simulink model "mode_glissant"  (R2016b)
settings: Solver=FixedStepAuto  StartTime=0.0  StopTime=10.0  FixedStep=.1  RelTol=1e-3
settings Model: Creator=vanou  LastModifiedBy=vanou

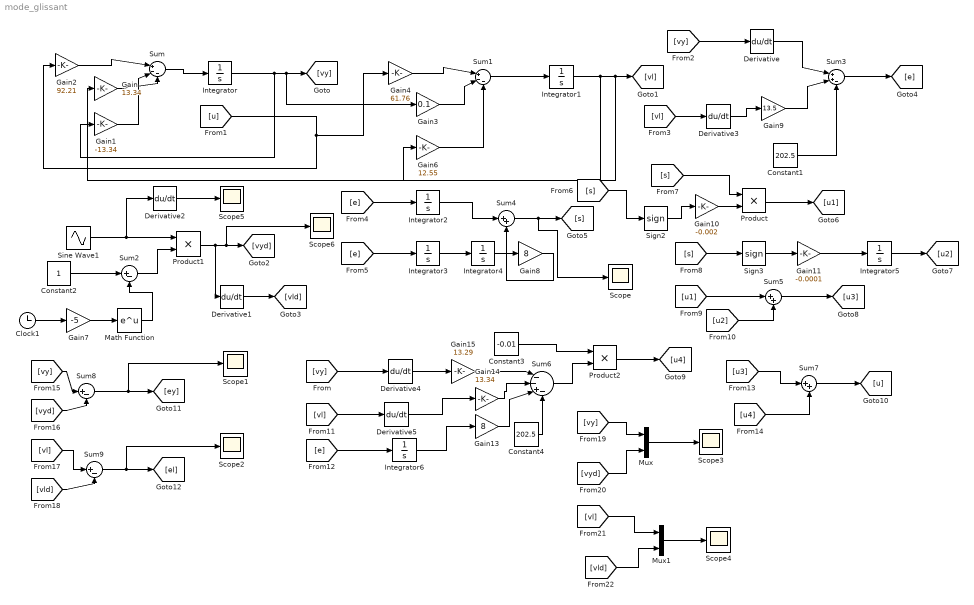
== system mode_glissant ==
  Clock1 : Clock
  Constant1 : Constant  Value=202.5
  Constant2 : Constant
  Constant3 : Constant  Value=-0.01
  Constant4 : Constant  Value=202.5
  Derivative{,1..5} (6 alike) : Derivative
  Gain : Gain  Gain=13.34
  Gain1 : Gain  Gain=-13.34
  Gain10 : Gain  Gain=-0.002
  Gain11 : Gain  Gain=-0.0001
  Gain13 : Gain  Gain=8
  Gain14 : Gain  Gain=13.34
  Gain15 : Gain  Gain=13.29
  Gain2 : Gain  Gain=92.21
  Gain3 : Gain  Gain=0.1
  Gain4 : Gain  Gain=61.76
  Gain6 : Gain  Gain=12.55
  Gain7 : Gain  Gain=-5
  Gain8 : Gain  Gain=8
  Gain9 : Gain  Gain=13.5
  Integrator{,1..6} (7 alike) : Integrator
  Math Function : Math  SaturateOnIntegerOverflow=on
  Mux : Mux  Inputs=2
  Mux1 : Mux  Inputs=2
  Product : Product
  Product1 : Product
  Product2 : Product
  Scope{,1..6} (7 alike) : Scope
  Sign2 : Signum
  Sign3 : Signum
  Sine Wave1 : Sin  SampleTime=0
  Sum : Sum  Inputs=|+--
  Sum1 : Sum  Inputs=|+--
  Sum2 : Sum  Inputs=|+-
  Sum3 : Sum  Inputs=|++-
  Sum4 : Sum  Inputs=|++
  Sum5 : Sum  Inputs=|++
  Sum6 : Sum  Inputs=|--+-
  Sum7 : Sum  Inputs=|++
  Sum8 : Sum  Inputs=|+-
  Sum9 : Sum  Inputs=|+-
  wires:
  Sum/1 -> Integrator/1
  Gain2/1 -> Sum/1
  Gain1/1 -> Sum/2
  Gain/1 -> Sum/3
  Sum1/1 -> Integrator1/1
  Gain4/1 -> Sum1/1
  Gain3/1 -> Sum1/2
  Integrator/1 -> Gain1/1, Gain3/1, [vy]
  [u] -> Gain2/1, Gain4/1
  Gain6/1 -> Sum1/3
  Integrator1/1 -> Gain6/1, Gain/1, [vl]
  Clock1/1 -> Gain7/1
  Gain7/1 -> Math Function/1
  Sine Wave1/1 -> Derivative2/1, Product1/1
  Math Function/1 -> Sum2/2
  Constant2/1 -> Sum2/1
  Sum2/1 -> Product1/2
  Product1/1 -> Derivative1/1, Scope6/1, [vyd]
  Derivative1/1 -> [vld]
  [vy] -> Derivative/1
  Derivative/1 -> Sum3/1
  [vl] -> Derivative3/1
  Gain9/1 -> Sum3/2
  Derivative3/1 -> Gain9/1
  Constant1/1 -> Sum3/3
  Sum3/1 -> [e]
  [e] -> Integrator2/1
  [e] -> Integrator3/1
  Integrator3/1 -> Integrator4/1
  Integrator2/1 -> Sum4/1
  Sum4/1 -> Scope/1, [s]
  Integrator4/1 -> Gain8/1
  Gain8/1 -> Sum4/2
  Product/1 -> [u1]
  [s] -> Sign2/1
  Sign2/1 -> Gain10/1
  Gain10/1 -> Product/2
  [s] -> Product/1
  [s] -> Sign3/1
  Sign3/1 -> Gain11/1
  Gain11/1 -> Integrator5/1
  Integrator5/1 -> [u2]
  [u1] -> Sum5/1
  [u2] -> Sum5/2
  Sum5/1 -> [u3]
  Product2/1 -> [u4]
  Constant3/1 -> Product2/1
  Sum6/1 -> Product2/2
  Gain15/1 -> Sum6/1
  Gain14/1 -> Sum6/2
  Gain13/1 -> Sum6/3
  Constant4/1 -> Sum6/4
  [vy] -> Derivative4/1
  Derivative4/1 -> Gain15/1
  [vl] -> Derivative5/1
  Derivative5/1 -> Gain14/1
  [e] -> Integrator6/1
  Integrator6/1 -> Gain13/1
  Sum7/1 -> [u]
  [u3] -> Sum7/1
  [u4] -> Sum7/2
  [vy] -> Sum8/1
  [vyd] -> Sum8/2
  [vl] -> Sum9/1
  [vld] -> Sum9/2
  Sum8/1 -> Scope1/1, [ey]
  Sum9/1 -> Scope2/1, [el]
  [vld] -> Mux1/2
  [vy] -> Mux/1
  [vyd] -> Mux/2
  Mux/1 -> Scope3/1
  Mux1/1 -> Scope4/1
  [vl] -> Mux1/1
  Derivative2/1 -> Scope5/1
